simulink model "disturbancesRough"  (R2018b)
settings: Solver=FixedStepAuto  StartTime=0.0  StopTime=6000  RelTol=1e-3
undefined symbols (not defined in the file): simParams
libraries: dspstat3 x12, vrlib x4, dspmathops x1, teme2eci_lib x1, clock_lib x1, time_Lib x1, aerolibutil x1, magField_lib x1, sgp4_lib_fsw x1
settings Model: Creator=Taylor  LastModifiedBy=Taylor

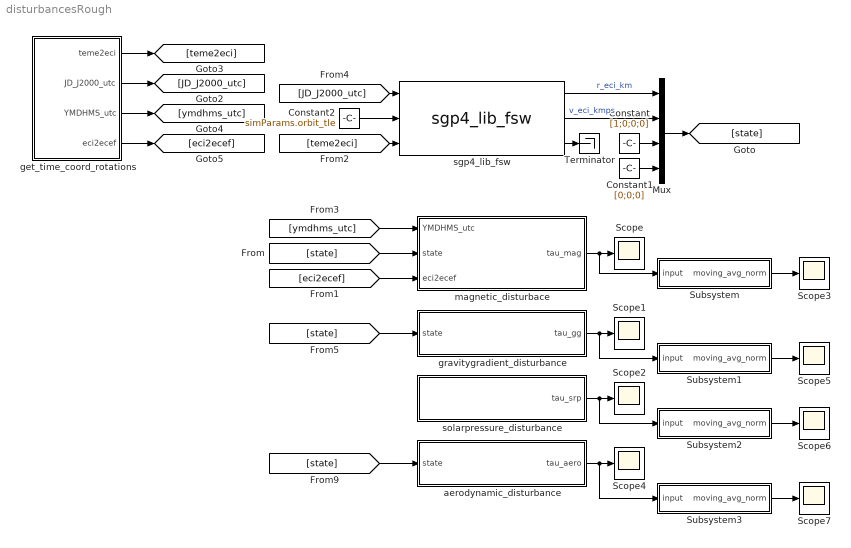
== system disturbancesRough ==
  Constant : Constant  Value=[1;0;0;0]
  Constant1 : Constant  Value=[0;0;0]
  Constant2 : Constant  Value=simParams.orbit_tle
  Mux : Mux  Inputs=[3 3 4 3]
  Scope{,1..7} (8 alike) : Scope
  Subsystem : Subsystem
  Subsystem1 : Subsystem
  Subsystem2 : Subsystem
  Subsystem3 : Subsystem
  Terminator : Terminator
  aerodynamic_disturbance : Subsystem
  get_time_coord_rotations : Subsystem
  gravitygradient_disturbance : Subsystem
  magnetic_disturbace : Subsystem
  sgp4_lib_fsw : sgp4_lib_fsw/sgp4_lib_fsw  SystemSampleTime=-1
  solarpressure_disturbance : Subsystem
  wires:
  get_time_coord_rotations/3(YMDHMS_utc) -> [ymdhms_utc]
  get_time_coord_rotations/1(teme2eci) -> [teme2eci]
  get_time_coord_rotations/4("eci2ecef ") -> [eci2ecef]
  get_time_coord_rotations/2(JD_J2000_utc) -> [JD_J2000_utc]
  Mux/1 -> [state]
  sgp4_lib_fsw/2 -> Mux/2  "v_eci_kmps"
  sgp4_lib_fsw/1 -> Mux/1  "r_eci_km"
  sgp4_lib_fsw/3 -> Terminator/1
  Constant/1 -> Mux/3
  Constant1/1 -> Mux/4
  [teme2eci] -> sgp4_lib_fsw/3
  [JD_J2000_utc] -> sgp4_lib_fsw/1
  Constant2/1 -> sgp4_lib_fsw/2
  [ymdhms_utc] -> magnetic_disturbace/1(YMDHMS_utc)
  [state] -> magnetic_disturbace/2(state)
  [eci2ecef] -> magnetic_disturbace/3(eci2ecef)
  magnetic_disturbace/1(tau_mag) -> Subsystem/1(input), Scope/1
  [state] -> gravitygradient_disturbance/1(state)
  gravitygradient_disturbance/1(tau_gg) -> Subsystem1/1(input), Scope1/1
  aerodynamic_disturbance/1(tau_aero) -> Subsystem3/1(input), Scope4/1
  [state] -> aerodynamic_disturbance/1(state)
  solarpressure_disturbance/1(tau_srp) -> Subsystem2/1(input), Scope2/1
  Subsystem/1(moving_avg_norm) -> Scope3/1
  Subsystem1/1(moving_avg_norm) -> Scope5/1
  Subsystem2/1(moving_avg_norm) -> Scope6/1
  Subsystem3/1(moving_avg_norm) -> Scope7/1

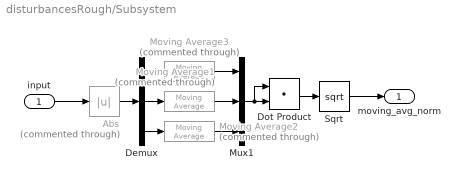
== system disturbancesRough/Subsystem ==
  input : Inport
  Abs : Abs  Commented=through
  Demux : Demux  Outputs=3
  Dot Product : DotProduct  InputSameDT=on  OutDataTypeStr=Inherit: Inherit via internal rule
  Moving Average1 : dspstat3/Moving Average  Commented=through  Method=Sliding window  ForgettingFactorPort=off  SpecifyWindowLength=off  WindowLength=4  ForgettingFactor=0.9  SimulateUsing=Code generation
  Moving Average2 : dspstat3/Moving Average  Commented=through  Method=Sliding window  ForgettingFactorPort=off  SpecifyWindowLength=off  WindowLength=4  ForgettingFactor=0.9  SimulateUsing=Code generation
  Moving Average3 : dspstat3/Moving Average  Commented=through  Method=Sliding window  ForgettingFactorPort=off  SpecifyWindowLength=off  WindowLength=4  ForgettingFactor=0.9  SimulateUsing=Code generation
  Mux1 : Mux  Inputs=3
  Sqrt : Sqrt  SaturateOnIntegerOverflow=on
  moving_avg_norm : Outport
  wires:
  input/1 -> Abs/1
  Dot Product/1 -> Sqrt/1
  Demux/1 -> Moving Average3/1
  Moving Average1/1 -> Mux1/2
  Moving Average3/1 -> Mux1/1
  Demux/3 -> Moving Average2/1
  Moving Average2/1 -> Mux1/3
  Demux/2 -> Moving Average1/1
  Sqrt/1 -> moving_avg_norm/1
  Abs/1 -> Demux/1
  Mux1/1 -> Dot Product/1, Dot Product/2

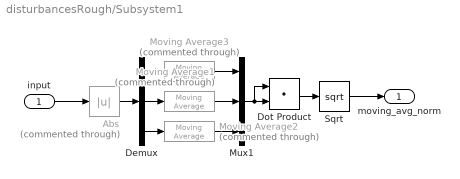
== system disturbancesRough/Subsystem1 ==
  input : Inport
  Abs : Abs  Commented=through
  Demux : Demux  Outputs=3
  Dot Product : DotProduct  InputSameDT=on  OutDataTypeStr=Inherit: Inherit via internal rule
  Moving Average1 : dspstat3/Moving Average  Commented=through  Method=Sliding window  ForgettingFactorPort=off  SpecifyWindowLength=off  WindowLength=4  ForgettingFactor=0.9  SimulateUsing=Code generation
  Moving Average2 : dspstat3/Moving Average  Commented=through  Method=Sliding window  ForgettingFactorPort=off  SpecifyWindowLength=off  WindowLength=4  ForgettingFactor=0.9  SimulateUsing=Code generation
  Moving Average3 : dspstat3/Moving Average  Commented=through  Method=Sliding window  ForgettingFactorPort=off  SpecifyWindowLength=off  WindowLength=4  ForgettingFactor=0.9  SimulateUsing=Code generation
  Mux1 : Mux  Inputs=3
  Sqrt : Sqrt  SaturateOnIntegerOverflow=on
  moving_avg_norm : Outport
  wires:
  Mux1/1 -> Dot Product/2, Dot Product/1
  Abs/1 -> Demux/1
  Sqrt/1 -> moving_avg_norm/1
  Demux/2 -> Moving Average1/1
  Moving Average2/1 -> Mux1/3
  Demux/3 -> Moving Average2/1
  Moving Average3/1 -> Mux1/1
  Moving Average1/1 -> Mux1/2
  Demux/1 -> Moving Average3/1
  Dot Product/1 -> Sqrt/1
  input/1 -> Abs/1

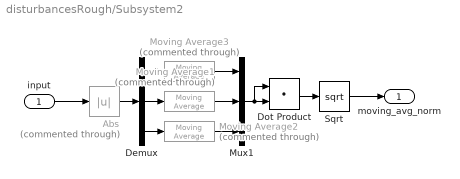
== system disturbancesRough/Subsystem2 ==
  input : Inport
  Abs : Abs  Commented=through
  Demux : Demux  Outputs=3
  Dot Product : DotProduct  InputSameDT=on  OutDataTypeStr=Inherit: Inherit via internal rule
  Moving Average1 : dspstat3/Moving Average  Commented=through  Method=Sliding window  ForgettingFactorPort=off  SpecifyWindowLength=off  WindowLength=4  ForgettingFactor=0.9  SimulateUsing=Code generation
  Moving Average2 : dspstat3/Moving Average  Commented=through  Method=Sliding window  ForgettingFactorPort=off  SpecifyWindowLength=off  WindowLength=4  ForgettingFactor=0.9  SimulateUsing=Code generation
  Moving Average3 : dspstat3/Moving Average  Commented=through  Method=Sliding window  ForgettingFactorPort=off  SpecifyWindowLength=off  WindowLength=4  ForgettingFactor=0.9  SimulateUsing=Code generation
  Mux1 : Mux  Inputs=3
  Sqrt : Sqrt  SaturateOnIntegerOverflow=on
  moving_avg_norm : Outport
  wires:
  input/1 -> Abs/1
  Dot Product/1 -> Sqrt/1
  Demux/1 -> Moving Average3/1
  Moving Average1/1 -> Mux1/2
  Moving Average3/1 -> Mux1/1
  Demux/3 -> Moving Average2/1
  Moving Average2/1 -> Mux1/3
  Demux/2 -> Moving Average1/1
  Sqrt/1 -> moving_avg_norm/1
  Abs/1 -> Demux/1
  Mux1/1 -> Dot Product/1, Dot Product/2

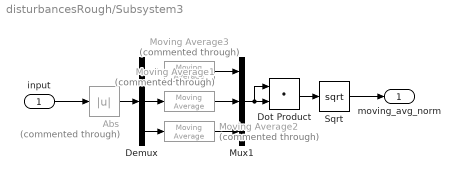
== system disturbancesRough/Subsystem3 ==
  input : Inport
  Abs : Abs  Commented=through
  Demux : Demux  Outputs=3
  Dot Product : DotProduct  InputSameDT=on  OutDataTypeStr=Inherit: Inherit via internal rule
  Moving Average1 : dspstat3/Moving Average  Commented=through  Method=Sliding window  ForgettingFactorPort=off  SpecifyWindowLength=off  WindowLength=4  ForgettingFactor=0.9  SimulateUsing=Code generation
  Moving Average2 : dspstat3/Moving Average  Commented=through  Method=Sliding window  ForgettingFactorPort=off  SpecifyWindowLength=off  WindowLength=4  ForgettingFactor=0.9  SimulateUsing=Code generation
  Moving Average3 : dspstat3/Moving Average  Commented=through  Method=Sliding window  ForgettingFactorPort=off  SpecifyWindowLength=off  WindowLength=4  ForgettingFactor=0.9  SimulateUsing=Code generation
  Mux1 : Mux  Inputs=3
  Sqrt : Sqrt  SaturateOnIntegerOverflow=on
  moving_avg_norm : Outport
  wires:
  Mux1/1 -> Dot Product/2, Dot Product/1
  Abs/1 -> Demux/1
  Sqrt/1 -> moving_avg_norm/1
  Demux/2 -> Moving Average1/1
  Moving Average2/1 -> Mux1/3
  Demux/3 -> Moving Average2/1
  Moving Average3/1 -> Mux1/1
  Moving Average1/1 -> Mux1/2
  Demux/1 -> Moving Average3/1
  Dot Product/1 -> Sqrt/1
  input/1 -> Abs/1

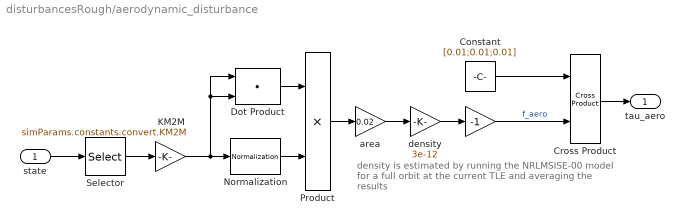
== system disturbancesRough/aerodynamic_disturbance ==
  note: density is estimated by running the NRLMSISE-00
      | model for a full orbit at the current TLE and averaging
      | the results
  state : Inport
  " " : Gain  Gain=-1
  Constant : Constant  Value=[0.01;0.01;0.01]
  Cross Product : vrlib/Utilities/Cross Product
      settings: SourceProductBaseCode=VR
  Dot Product : DotProduct  InputSameDT=on  OutDataTypeStr=Inherit: Inherit via internal rule
  KM2M : Gain  Gain=simParams.constants.convert.KM2M
  Normalization : dspmathops/Normalization  NormType=2-norm  Bias=1e-10  NormOver=Each column  Dimension=1  roundingMode=Floor  overflowMode=off  accumDataTypeStr=Inherit: Same as product output  accumLastDataTypeStr=Inherit: Same as product output  outputDataTypeStr=Inherit: Same as product output  outputMin=[]  outputMax=[]  outputLastDataTypeStr=Inherit: Same as product output
      settings: SourceProductName=DSP System Toolbox
  Product : Product
  Selector : Selector  InputPortWidth=13  IndexOptions=Index vector (dialog)  Indices=simParams.constants.id_v  OutputSizes=1
  area : Gain  Gain=0.02
  density : Gain  Gain=3e-12
  tau_aero : Outport
  wires:
  state/1 -> Selector/1
  Selector/1 -> KM2M/1
  Normalization/1 -> Product/2
  Dot Product/1 -> Product/1
  Product/1 -> area/1
  area/1 -> density/1
  density/1 -> " "/1
  " "/1 -> Cross Product/2  "f_aero"
  Constant/1 -> Cross Product/1
  Cross Product/1 -> tau_aero/1
  KM2M/1 -> Dot Product/1, Dot Product/2, Normalization/1

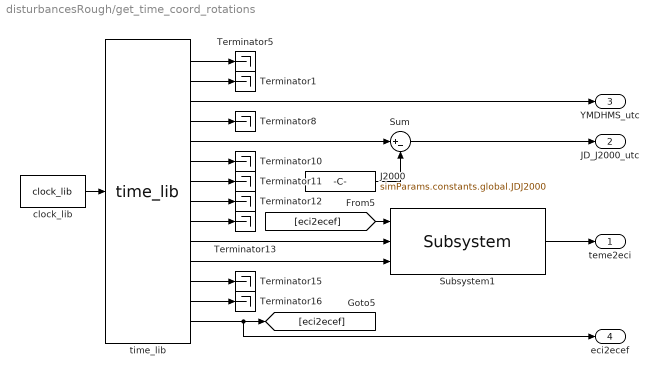
== system disturbancesRough/get_time_coord_rotations ==
  J2000 : Constant  Value=simParams.constants.global.JDJ2000  OutDataTypeStr=Inherit: Inherit via back propagation
  Subsystem1 : teme2eci_lib/Subsystem  SystemSampleTime=-1
  Sum : Sum  Inputs=|+-
  Terminator{1,5,8,10..13,15..16} (9 alike) : Terminator
  clock_lib : clock_lib/clock_lib  SystemSampleTime=-1
  "time_lib " : time_Lib/time_lib    SystemSampleTime=-1
  teme2eci : Outport
  JD_J2000_utc : Outport  Port=2
  YMDHMS_utc : Outport  Port=3
  "eci2ecef " : Outport  Port=4
  wires:
  "time_lib "/11 -> Subsystem1/3
  [eci2ecef] -> Subsystem1/1
  J2000/1 -> Sum/2
  "time_lib "/10 -> Subsystem1/2
  "time_lib "/6 -> Terminator10/1
  "time_lib "/13 -> Terminator16/1
  clock_lib/1 -> "time_lib "/1
  "time_lib "/3 -> YMDHMS_utc/1
  "time_lib "/7 -> Terminator11/1
  "time_lib "/2 -> Terminator1/1
  "time_lib "/5 -> Sum/1
  "time_lib "/14 -> "eci2ecef "/1, [eci2ecef]
  "time_lib "/12 -> Terminator15/1
  "time_lib "/1 -> Terminator5/1
  "time_lib "/4 -> Terminator8/1
  "time_lib "/8 -> Terminator12/1
  "time_lib "/9 -> Terminator13/1
  Subsystem1/1 -> teme2eci/1
  Sum/1 -> JD_J2000_utc/1

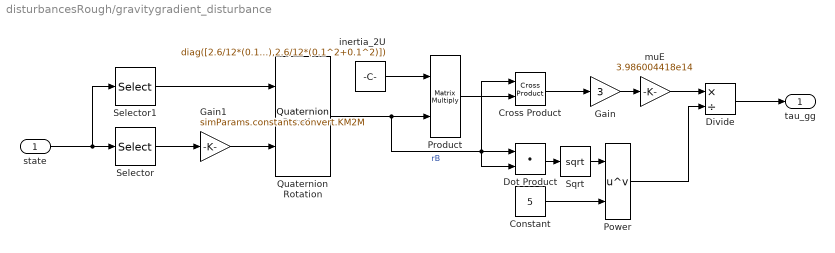
== system disturbancesRough/gravitygradient_disturbance ==
  state : Inport
  Constant : Constant  Value=5
  Cross Product : vrlib/Utilities/Cross Product
      settings: SourceProductBaseCode=VR
  Divide : Product  Inputs=*/
  Dot Product : DotProduct  InputSameDT=on  OutDataTypeStr=Inherit: Inherit via internal rule
  Gain : Gain  Gain=3
  Gain1 : Gain  Gain=simParams.constants.convert.KM2M
  Power : Math  Operator=pow  SaturateOnIntegerOverflow=on
  Product : Product  Multiplication=Matrix(*)
  Quaternion Rotation : aerolibutil/Quaternion Rotation
  Selector : Selector  InputPortWidth=13  IndexOptions=Index vector (dialog)  Indices=fswParams.constants.id_r  OutputSizes=1
  Selector1 : Selector  InputPortWidth=13  IndexOptions=Index vector (dialog)  Indices=fswParams.constants.id_q  OutputSizes=1
  Sqrt : Sqrt  SaturateOnIntegerOverflow=on
  inertia_2U : Constant  Value=diag([2.6/12*(0.1^2+0.2^2),2.6/12*(0.1^2+0.2^2),2.6/12*(0.1^2+0.1^2)])
  muE : Gain  Gain=3.986004418e14
  tau_gg : Outport
  wires:
  state/1 -> Selector1/1, Selector/1
  Selector/1 -> Gain1/1
  Selector1/1 -> Quaternion Rotation/1
  inertia_2U/1 -> Product/1
  Quaternion Rotation/1 -> Dot Product/2, Dot Product/1, Cross Product/1, Product/2  "rB"
  Product/1 -> Cross Product/2
  Cross Product/1 -> Gain/1
  Dot Product/1 -> Sqrt/1
  Constant/1 -> Power/2
  Sqrt/1 -> Power/1
  Gain/1 -> muE/1
  Power/1 -> Divide/2
  muE/1 -> Divide/1
  Divide/1 -> tau_gg/1
  Gain1/1 -> Quaternion Rotation/2

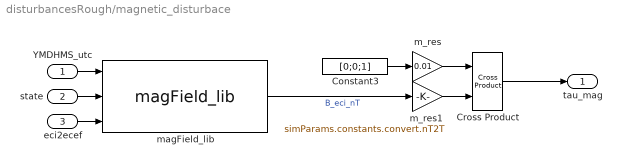
== system disturbancesRough/magnetic_disturbace ==
  YMDHMS_utc : Inport
  state : Inport  Port=2
  eci2ecef : Inport  Port=3
  Constant3 : Constant  Value=[0;0;1]
  Cross Product : vrlib/Utilities/Cross Product
      settings: SourceProductBaseCode=VR
  m_res : Gain  Gain=0.01
  m_res1 : Gain  Gain=simParams.constants.convert.nT2T
  magField_lib : magField_lib/magField_lib  SystemSampleTime=-1
  tau_mag : Outport
  wires:
  Cross Product/1 -> tau_mag/1
  state/1 -> magField_lib/2
  eci2ecef/1 -> magField_lib/3
  m_res1/1 -> Cross Product/2
  Constant3/1 -> m_res/1
  magField_lib/1 -> m_res1/1  "B_eci_nT"
  YMDHMS_utc/1 -> magField_lib/1
  m_res/1 -> Cross Product/1

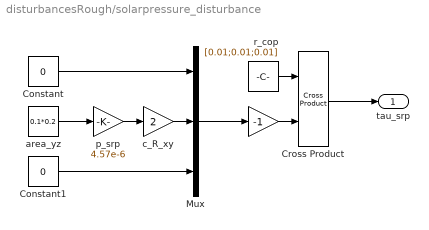
== system disturbancesRough/solarpressure_disturbance ==
  " " : Gain  Gain=-1
  Constant : Constant  Value=0
  Constant1 : Constant  Value=0
  Cross Product : vrlib/Utilities/Cross Product
      settings: SourceProductBaseCode=VR
  Mux : Mux  Inputs=3
  area_yz : Constant  Value=0.1*0.2
  c_R_xy : Gain  Gain=2
  p_srp : Gain  Gain=4.57e-6
  "r_cop " : Constant  Value=[0.01;0.01;0.01]
  tau_srp : Outport
  wires:
  area_yz/1 -> p_srp/1
  p_srp/1 -> c_R_xy/1
  c_R_xy/1 -> Mux/2
  Constant1/1 -> Mux/3
  Constant/1 -> Mux/1
  Mux/1 -> " "/1
  "r_cop "/1 -> Cross Product/1
  Cross Product/1 -> tau_srp/1
  " "/1 -> Cross Product/2
